simulink model "Panneau_PV_avec_charge_variable"  (R2017b)
settings: Solver=VariableStepAuto  StartTime=0.0  StopTime=inf  FixedStep=1e-8  MinStep=1e-8  RelTol=1e-3
InitFcn:
  | fig_h = figure;
  | ax_h = axes;
  | set(ax_h,'Xlim',[0 22],'YLim',[0 0.3])
libraries: fl_lib x4, nesl_utility x3, Library_SII x2, elec_lib x1, simulink x1
settings Model: Creator=Cedrick  LastModifiedBy=Cedrick

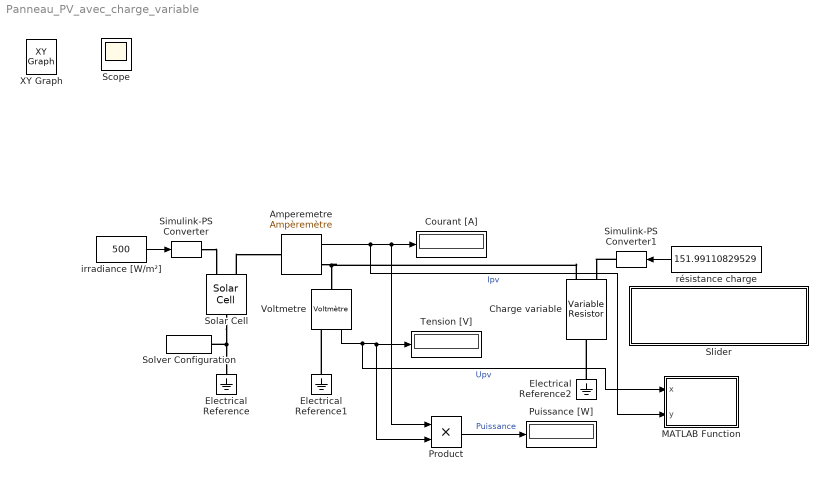
== system Panneau_PV_avec_charge_variable ==
  Amperemetre : Library_SII/Electronique/Ampèremètre
      settings: SourceProductName=SII
  Charge variable : fl_lib/Electrical/Electrical Elements/Variable Resistor  Rmin=1 Ohm  i_specify=off  i_priority=None  i=0 A  i_nominal_specify=off  i_nominal_unit=A  i_nominal_value=1  v_specify=off  v_priority=None  v=0 V  v_nominal_specify=off  v_nominal_unit=V  v_nominal_value=1
  Courant [A] : Display
  Electrical Reference : fl_lib/Electrical/Electrical Elements/Electrical Reference
  Electrical Reference1 : fl_lib/Electrical/Electrical Elements/Electrical Reference
  Electrical Reference2 : fl_lib/Electrical/Electrical Elements/Electrical Reference
  MATLAB Function : MATLAB Function  TreatAsAtomicUnit=on  SystemSampleTime=10
  Product : Product
  Puissance [W] : Display
  Simulink-PS Converter : nesl_utility/Simulink-PS Converter  PhysicalDomain=network_engine_domain  SubClassName=ps_input  LeftPortType=input  RightPortType=output  PseudoPeriodic=off  Frequencies=[]  NoiseDistribution=none  NoiseParameters=[]  Unit=1  AffineConversion=off  FilteringAndDerivatives=provide  SimscapeFilterOrder=1  InputFilterTimeConstant=0.001  UdotUserProvided=0
  Simulink-PS Converter1 : nesl_utility/Simulink-PS Converter  PhysicalDomain=network_engine_domain  SubClassName=ps_input  LeftPortType=input  RightPortType=output  PseudoPeriodic=off  Frequencies=[]  NoiseDistribution=none  NoiseParameters=[]  Unit=1  AffineConversion=off  FilteringAndDerivatives=provide  SimscapeFilterOrder=1  InputFilterTimeConstant=0.001  UdotUserProvided=0
  Slider : Subsystem  DialogController=hmiCreateDDGDialog  IsWebBlock=on  mask(MWDashboardBlock){webBlockId=574ab3c5-b9e4-429a-9142-107109e8eed0, webBlockType=slider, ShowInLibBrowser=on, ShowInitialText=on, HMISrcModelName=ChargeurSolaire}
      mask prompts: webBlockId "WebBlock Id"; webBlockType "WebBlock Type"; HMISrcModelName "Source Model"
      mask help: SimulinkHMI:dialogs:SliderDialogDesc
      mask Help: helpview([docroot '/mapfiles/simulink.map'], 'hmi_slider')
      mask Display:
      | if strcmp(get_param(bdroot(gcb),'BlockDiagramType'), 'library')
      |     image([(matlabroot) '/toolbox/simulink/hmi/icons/Slider.png']);
      | end
  Solar Cell : elec_lib/Sources/Solar Cell  prm=1  Isc=0.32 A  Voc=0.6 V  Is=1e-6 A  Is2=0 A  Iph=7.34 A  Ir0=1000 W/m^2  ec=1.5  N2=2  Rs=0 Ohm  Rp=inf Ohm  N_series=36  TIPH1=0 1/K  EG=1.11 eV  TXIS1=3  TXIS2=3  TRS1=0  TRP1=0  Tmeas=25 degC  TFIXED=25 degC  thermal_mass=100 J/K  initial_temperature=25 degC
      settings: SourceProductName=Simscape Electronics  SourceProductBaseCode=SN
  Solver Configuration : nesl_utility/Solver Configuration  PhysicalDomain=network_engine_domain  SubClassName=solver  LeftPortType=input  RightPortType=generic  Accelerate=off  Tones=[]  Harmonics=[]  SimulateNoise=off  Profile=off  UseLocalSampling=off  EnableSwitchedLinearOptims=on  FrequencyDomain=off  UseCCode=off  RelTol=0.001  AbsTol=1e-06  MinStep=1e-09  ToWorkspace=off  RevertToSquareIcSolve=off  NumHomotopyIterations=100  PhasorMode=off  PhasorModeNumHarmonics=1  DoDC=off  ResidualTolerance=1e-09  UseLocalSolver=off  LocalSolverChoice=NE_BACKWARD_EULER_ADVANCER  LocalSolverSampleTime=0.001  DoFixedCost=off  MaxNonlinIter=3  MaxModeIter=2  LinearAlgebra=Sparse  DelaysMemoryBudget=1024  AutomaticFiltering=on  FilteringTimeConstant=0.001
  Tension [V] : Display
  Voltmetre : Library_SII/Electronique/Voltmètre
      settings: SourceProductName=SII
  irradiance [W/m²] : Constant  Value=500
  résistance charge : Constant  Value=151.99110829529
  Scope : Scope
  XY Graph : simulink/Sinks/XY Graph  IOType=viewer  xmin=0  xmax=22  ymin=0  ymax=0.3  st=10
  wires:
  irradiance [W/m²]/1 -> Simulink-PS Converter/1
  Amperemetre/1 -> MATLAB Function/2(y), Product/1, Courant [A]/1  "Ipv"
  Voltmetre/1 -> MATLAB Function/1(x), Tension [V]/1, Product/2  "Upv"
  résistance charge/1 -> Simulink-PS Converter1/1
  Product/1 -> Puissance [W]/1  "Puissance"
  connections:
  Solar Cell/RConn1 -- Solver Configuration/RConn1 -- Electrical Reference/LConn1
  Electrical Reference1/LConn1 -- Voltmetre/RConn1
  Simulink-PS Converter/RConn1 -- Solar Cell/LConn1
  Solar Cell/LConn2 -- Amperemetre/LConn1
  Amperemetre/RConn1 -- Charge variable/LConn2 -- Voltmetre/LConn1
  Simulink-PS Converter1/RConn1 -- Charge variable/LConn1
  Electrical Reference2/LConn1 -- Charge variable/RConn1

== system Panneau_PV_avec_charge_variable/Slider ==

== matlab function Panneau_PV_avec_charge_variable/MATLAB Function ==
  data: x input; y input
function fcn(x, y)
coder.extrinsic('plot')
plot(x,y,'-o','Markersize',6,'MarkerFaceColor','g');
hold on;
set(gca,'XLim',[0 22],'Ylim',[0 0.3])
